simulink model "TST_CEngDsT_VD"  (R2016b)
settings: Solver=FixedStepDiscrete  StartTime=0.0  StopTime=simTime  FixedStep=sampleTime  RelTol=1e-3
values from neighbouring files (symbols this model uses):
  testCase = 1    [initTST_CEngDsT_VD_001.m]    (also in initTST_CEngDsT_VD_002.m = 2; initTST_CEngDsT_VD_003.m = 3; initTST_CEngDsT_VD_004.m = 4)
libraries: simulink x9, UnitTest_Lib x6
settings Model: Creator=dulinggang  LastModifiedBy=dulinggang
settings DebuggingCC: SignalRangeChecking=error

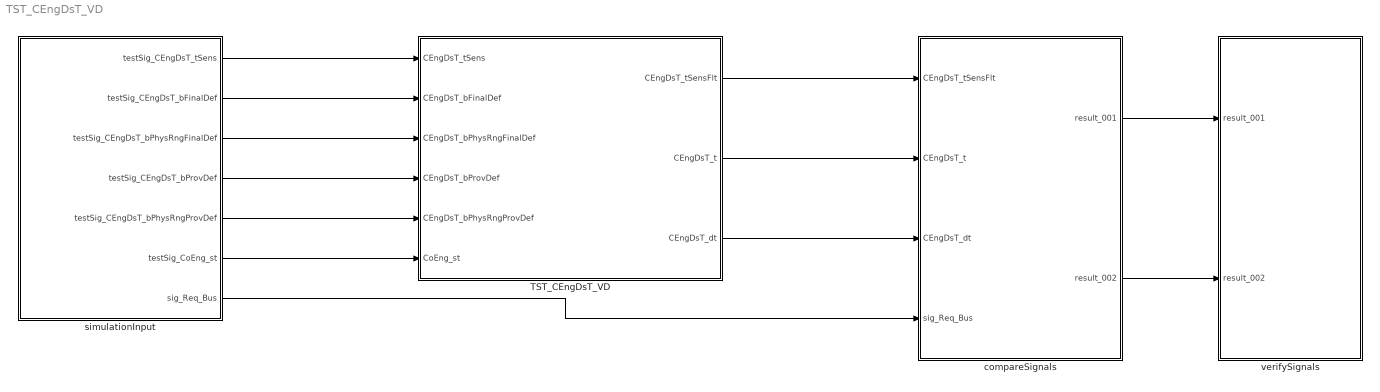
== system TST_CEngDsT_VD ==
  TST_CEngDsT_VD : Subsystem
  compareSignals : Subsystem
  simulationInput : Subsystem
  verifySignals : Subsystem
  wires:
  simulationInput/1(testSig_CEngDsT_tSens) -> TST_CEngDsT_VD/1(CEngDsT_tSens)
  simulationInput/2(testSig_CEngDsT_bFinalDef) -> TST_CEngDsT_VD/2(CEngDsT_bFinalDef)
  simulationInput/3(testSig_CEngDsT_bPhysRngFinalDef) -> TST_CEngDsT_VD/3(CEngDsT_bPhysRngFinalDef)
  simulationInput/4(testSig_CEngDsT_bProvDef) -> TST_CEngDsT_VD/4(CEngDsT_bProvDef)
  simulationInput/5(testSig_CEngDsT_bPhysRngProvDef) -> TST_CEngDsT_VD/5(CEngDsT_bPhysRngProvDef)
  simulationInput/6(testSig_CoEng_st) -> TST_CEngDsT_VD/6(CoEng_st)
  TST_CEngDsT_VD/1(CEngDsT_tSensFlt) -> compareSignals/1(CEngDsT_tSensFlt)
  TST_CEngDsT_VD/2(CEngDsT_t) -> compareSignals/2(CEngDsT_t)
  TST_CEngDsT_VD/3(CEngDsT_dt) -> compareSignals/3(CEngDsT_dt)
  simulationInput/7(sig_Req_Bus) -> compareSignals/4(sig_Req_Bus)
  compareSignals/1(result_001) -> verifySignals/1(result_001)
  compareSignals/2(result_002) -> verifySignals/2(result_002)

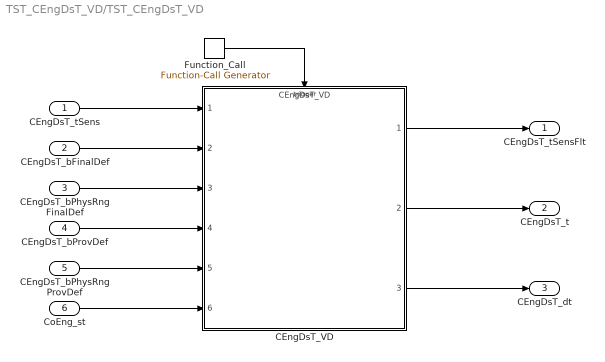
== system TST_CEngDsT_VD/TST_CEngDsT_VD ==
  CEngDsT_tSens : Inport
  CEngDsT_bFinalDef : Inport  Port=2
  CEngDsT_bPhysRngFinalDef : Inport  Port=3
  CEngDsT_bProvDef : Inport  Port=4
  CEngDsT_bPhysRngProvDef : Inport  Port=5
  CoEng_st : Inport  Port=6
  CEngDsT_VD : ModelReference  ModelNameDialog=CEngDsT_VD  SimulationMode=Normal  ModelReferenceVersion=1.125  TriggerPortName=function  TriggerPortTriggerType=function-call  TriggerPortStatesWhenEnabling=held
  Function_Call : simulink/Ports & Subsystems/Function-Call Generator  sample_time=sampleTime  numberOfIterations=1
  CEngDsT_tSensFlt : Outport
  CEngDsT_t : Outport  Port=2
  CEngDsT_dt : Outport  Port=3
  wires:
  Function_Call/1 -> CEngDsT_VD/Trigger
  CEngDsT_tSens/1 -> CEngDsT_VD/1
  CEngDsT_bFinalDef/1 -> CEngDsT_VD/2
  CEngDsT_bPhysRngFinalDef/1 -> CEngDsT_VD/3
  CEngDsT_bProvDef/1 -> CEngDsT_VD/4
  CEngDsT_bPhysRngProvDef/1 -> CEngDsT_VD/5
  CoEng_st/1 -> CEngDsT_VD/6
  CEngDsT_VD/1 -> CEngDsT_tSensFlt/1
  CEngDsT_VD/2 -> CEngDsT_t/1
  CEngDsT_VD/3 -> CEngDsT_dt/1

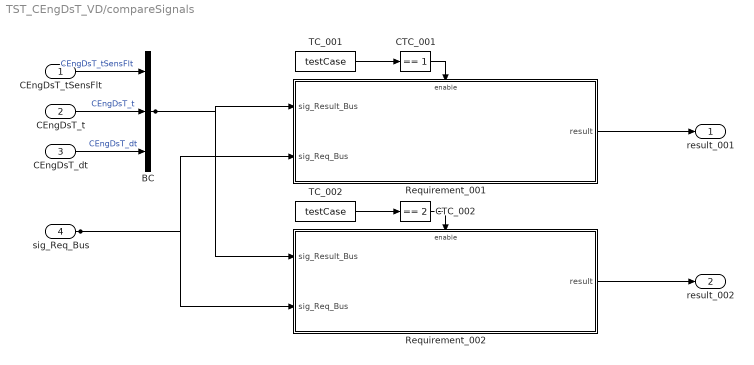
== system TST_CEngDsT_VD/compareSignals ==
  CEngDsT_tSensFlt : Inport
  CEngDsT_t : Inport  Port=2
  CEngDsT_dt : Inport  Port=3
  sig_Req_Bus : Inport  Port=4
  BC : BusCreator  Inputs=3
  CTC_001 : simulink/Logic and Bit Operations/Compare To Constant  relop===  const=1  OutDataTypeStr=boolean
  CTC_002 : simulink/Logic and Bit Operations/Compare To Constant  relop===  const=2  OutDataTypeStr=boolean
  Requirement_001 : Subsystem
  Requirement_002 : Subsystem
  TC_001 : Constant  Value=testCase
  TC_002 : Constant  Value=testCase
  result_001 : Outport
  result_002 : Outport  Port=2
  wires:
  CEngDsT_tSensFlt/1 -> BC/1  "CEngDsT_tSensFlt"
  CEngDsT_t/1 -> BC/2  "CEngDsT_t"
  CEngDsT_dt/1 -> BC/3  "CEngDsT_dt"
  TC_001/1 -> CTC_001/1
  CTC_001/1 -> Requirement_001/Enable
  sig_Req_Bus/1 -> Requirement_001/2(sig_Req_Bus), Requirement_002/2(sig_Req_Bus)
  BC/1 -> Requirement_001/1(sig_Result_Bus), Requirement_002/1(sig_Result_Bus)
  Requirement_001/1(result) -> result_001/1
  TC_002/1 -> CTC_002/1
  CTC_002/1 -> Requirement_002/Enable
  Requirement_002/1(result) -> result_002/1

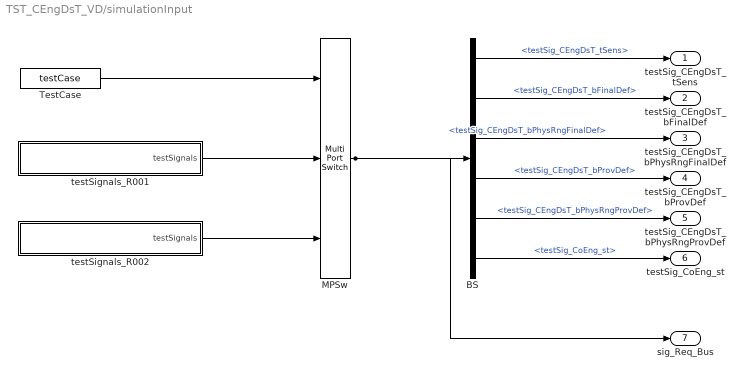
== system TST_CEngDsT_VD/simulationInput ==
  BS : BusSelector  OutputSignals=testSig_CEngDsT_tSens,testSig_CEngDsT_bFinalDef,testSig_CEngDsT_bPhysRngFinalDef,testSig_CEngDsT_bProvDef,testSig_CEngDsT_bPhysRngProvDef,testSig_CoEng_st
  MPSw : MultiPortSwitch  Inputs=2  SaturateOnIntegerOverflow=on  InputSameDT=on
  TestCase : Constant  Value=testCase
  testSignals_R001 : Subsystem
  testSignals_R002 : Subsystem
  testSig_CEngDsT_tSens : Outport
  testSig_CEngDsT_bFinalDef : Outport  Port=2
  testSig_CEngDsT_bPhysRngFinalDef : Outport  Port=3
  testSig_CEngDsT_bProvDef : Outport  Port=4
  testSig_CEngDsT_bPhysRngProvDef : Outport  Port=5
  testSig_CoEng_st : Outport  Port=6
  sig_Req_Bus : Outport  Port=7
  wires:
  BS/1 -> testSig_CEngDsT_tSens/1  "<testSig_CEngDsT_tSens>"
  BS/2 -> testSig_CEngDsT_bFinalDef/1  "<testSig_CEngDsT_bFinalDef>"
  BS/3 -> testSig_CEngDsT_bPhysRngFinalDef/1  "<testSig_CEngDsT_bPhysRngFinalDef>"
  BS/4 -> testSig_CEngDsT_bProvDef/1  "<testSig_CEngDsT_bProvDef>"
  BS/5 -> testSig_CEngDsT_bPhysRngProvDef/1  "<testSig_CEngDsT_bPhysRngProvDef>"
  BS/6 -> testSig_CoEng_st/1  "<testSig_CoEng_st>"
  MPSw/1 -> BS/1, sig_Req_Bus/1
  TestCase/1 -> MPSw/1
  testSignals_R001/1(testSignals) -> MPSw/2
  testSignals_R002/1(testSignals) -> MPSw/3

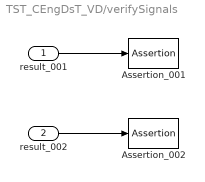
== system TST_CEngDsT_VD/verifySignals ==
  result_001 : Inport
  result_002 : Inport  Port=2
  Assertion_001 : Assertion  Enabled=off
  Assertion_002 : Assertion  Enabled=off
  wires:
  result_001/1 -> Assertion_001/1
  result_002/1 -> Assertion_002/1

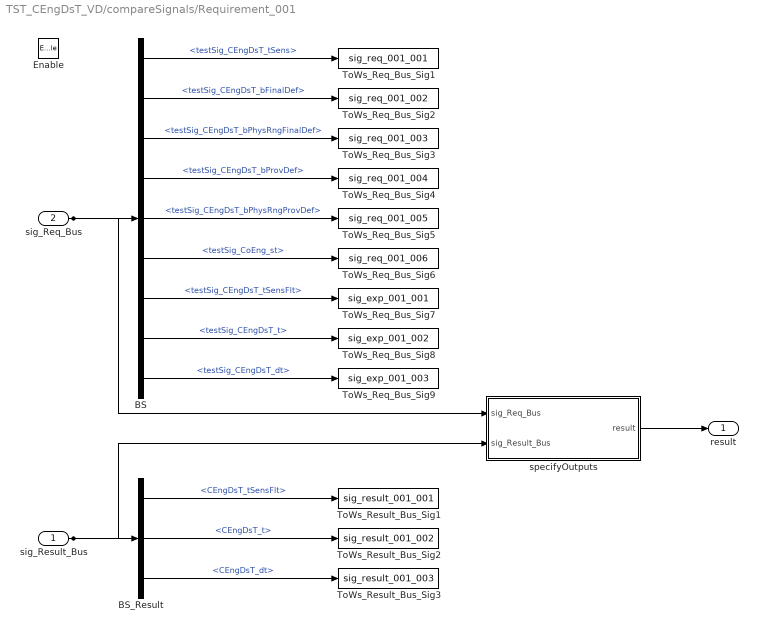
== system TST_CEngDsT_VD/compareSignals/Requirement_001 ==
  sig_Result_Bus : Inport
  sig_Req_Bus : Inport  Port=2
  Enable : EnablePort
  BS : BusSelector  OutputSignals=testSig_CEngDsT_tSens,testSig_CEngDsT_bFinalDef,testSig_CEngDsT_bPhysRngFinalDef,testSig_CEngDsT_bProvDef,testSig_CEngDsT_bPhysRngProvDef,testSig_CoEng_st,testSig_CEngDsT_tSensFlt,testSig_CEngDsT_t,testSig_CEngDsT_dt
  BS_Result : BusSelector  OutputSignals=CEngDsT_tSensFlt,CEngDsT_t,CEngDsT_dt
  ToWs_Req_Bus_Sig1 : ToWorkspace  VariableName=sig_req_001_001  SaveFormat=Structure With Time
  ToWs_Req_Bus_Sig2 : ToWorkspace  VariableName=sig_req_001_002  SaveFormat=Structure With Time
  ToWs_Req_Bus_Sig3 : ToWorkspace  VariableName=sig_req_001_003  SaveFormat=Structure With Time
  ToWs_Req_Bus_Sig4 : ToWorkspace  VariableName=sig_req_001_004  SaveFormat=Structure With Time
  ToWs_Req_Bus_Sig5 : ToWorkspace  VariableName=sig_req_001_005  SaveFormat=Structure With Time
  ToWs_Req_Bus_Sig6 : ToWorkspace  VariableName=sig_req_001_006  SaveFormat=Structure With Time
  ToWs_Req_Bus_Sig7 : ToWorkspace  VariableName=sig_exp_001_001  SaveFormat=Structure With Time
  ToWs_Req_Bus_Sig8 : ToWorkspace  VariableName=sig_exp_001_002  SaveFormat=Structure With Time
  ToWs_Req_Bus_Sig9 : ToWorkspace  VariableName=sig_exp_001_003  SaveFormat=Structure With Time
  ToWs_Result_Bus_Sig1 : ToWorkspace  VariableName=sig_result_001_001  SaveFormat=Structure With Time
  ToWs_Result_Bus_Sig2 : ToWorkspace  VariableName=sig_result_001_002  SaveFormat=Structure With Time
  ToWs_Result_Bus_Sig3 : ToWorkspace  VariableName=sig_result_001_003  SaveFormat=Structure With Time
  specifyOutputs : Subsystem
  result : Outport
  wires:
  sig_Req_Bus/1 -> BS/1, specifyOutputs/1(sig_Req_Bus)
  BS/1 -> ToWs_Req_Bus_Sig1/1  "<testSig_CEngDsT_tSens>"
  BS/2 -> ToWs_Req_Bus_Sig2/1  "<testSig_CEngDsT_bFinalDef>"
  BS/3 -> ToWs_Req_Bus_Sig3/1  "<testSig_CEngDsT_bPhysRngFinalDef>"
  BS/4 -> ToWs_Req_Bus_Sig4/1  "<testSig_CEngDsT_bProvDef>"
  BS/5 -> ToWs_Req_Bus_Sig5/1  "<testSig_CEngDsT_bPhysRngProvDef>"
  BS/6 -> ToWs_Req_Bus_Sig6/1  "<testSig_CoEng_st>"
  BS/7 -> ToWs_Req_Bus_Sig7/1  "<testSig_CEngDsT_tSensFlt>"
  BS/8 -> ToWs_Req_Bus_Sig8/1  "<testSig_CEngDsT_t>"
  BS/9 -> ToWs_Req_Bus_Sig9/1  "<testSig_CEngDsT_dt>"
  sig_Result_Bus/1 -> BS_Result/1, specifyOutputs/2(sig_Result_Bus)
  BS_Result/1 -> ToWs_Result_Bus_Sig1/1  "<CEngDsT_tSensFlt>"
  BS_Result/2 -> ToWs_Result_Bus_Sig2/1  "<CEngDsT_t>"
  BS_Result/3 -> ToWs_Result_Bus_Sig3/1  "<CEngDsT_dt>"
  specifyOutputs/1(result) -> result/1

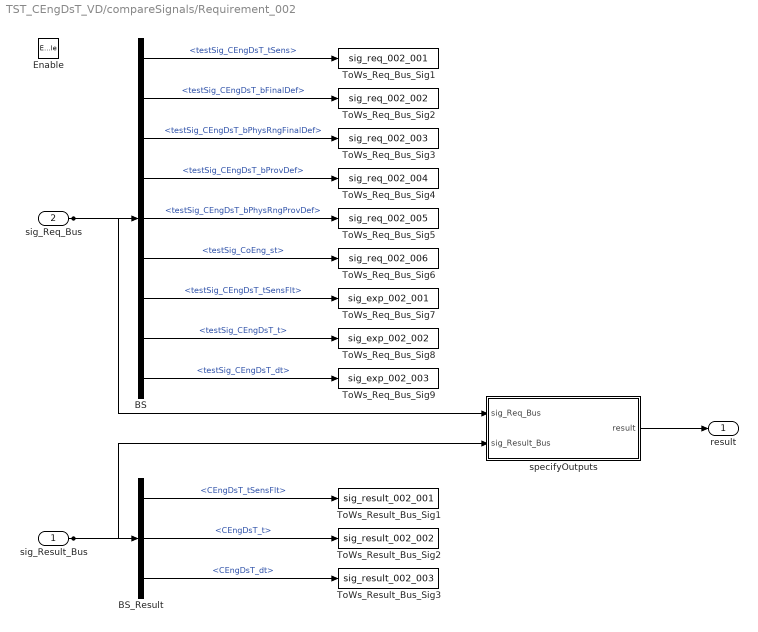
== system TST_CEngDsT_VD/compareSignals/Requirement_002 ==
  sig_Result_Bus : Inport
  sig_Req_Bus : Inport  Port=2
  Enable : EnablePort
  BS : BusSelector  OutputSignals=testSig_CEngDsT_tSens,testSig_CEngDsT_bFinalDef,testSig_CEngDsT_bPhysRngFinalDef,testSig_CEngDsT_bProvDef,testSig_CEngDsT_bPhysRngProvDef,testSig_CoEng_st,testSig_CEngDsT_tSensFlt,testSig_CEngDsT_t,testSig_CEngDsT_dt
  BS_Result : BusSelector  OutputSignals=CEngDsT_tSensFlt,CEngDsT_t,CEngDsT_dt
  ToWs_Req_Bus_Sig1 : ToWorkspace  VariableName=sig_req_002_001  SaveFormat=Structure With Time
  ToWs_Req_Bus_Sig2 : ToWorkspace  VariableName=sig_req_002_002  SaveFormat=Structure With Time
  ToWs_Req_Bus_Sig3 : ToWorkspace  VariableName=sig_req_002_003  SaveFormat=Structure With Time
  ToWs_Req_Bus_Sig4 : ToWorkspace  VariableName=sig_req_002_004  SaveFormat=Structure With Time
  ToWs_Req_Bus_Sig5 : ToWorkspace  VariableName=sig_req_002_005  SaveFormat=Structure With Time
  ToWs_Req_Bus_Sig6 : ToWorkspace  VariableName=sig_req_002_006  SaveFormat=Structure With Time
  ToWs_Req_Bus_Sig7 : ToWorkspace  VariableName=sig_exp_002_001  SaveFormat=Structure With Time
  ToWs_Req_Bus_Sig8 : ToWorkspace  VariableName=sig_exp_002_002  SaveFormat=Structure With Time
  ToWs_Req_Bus_Sig9 : ToWorkspace  VariableName=sig_exp_002_003  SaveFormat=Structure With Time
  ToWs_Result_Bus_Sig1 : ToWorkspace  VariableName=sig_result_002_001  SaveFormat=Structure With Time
  ToWs_Result_Bus_Sig2 : ToWorkspace  VariableName=sig_result_002_002  SaveFormat=Structure With Time
  ToWs_Result_Bus_Sig3 : ToWorkspace  VariableName=sig_result_002_003  SaveFormat=Structure With Time
  specifyOutputs : Subsystem
  result : Outport
  wires:
  sig_Req_Bus/1 -> BS/1, specifyOutputs/1(sig_Req_Bus)
  BS/1 -> ToWs_Req_Bus_Sig1/1  "<testSig_CEngDsT_tSens>"
  BS/2 -> ToWs_Req_Bus_Sig2/1  "<testSig_CEngDsT_bFinalDef>"
  BS/3 -> ToWs_Req_Bus_Sig3/1  "<testSig_CEngDsT_bPhysRngFinalDef>"
  BS/4 -> ToWs_Req_Bus_Sig4/1  "<testSig_CEngDsT_bProvDef>"
  BS/5 -> ToWs_Req_Bus_Sig5/1  "<testSig_CEngDsT_bPhysRngProvDef>"
  BS/6 -> ToWs_Req_Bus_Sig6/1  "<testSig_CoEng_st>"
  BS/7 -> ToWs_Req_Bus_Sig7/1  "<testSig_CEngDsT_tSensFlt>"
  BS/8 -> ToWs_Req_Bus_Sig8/1  "<testSig_CEngDsT_t>"
  BS/9 -> ToWs_Req_Bus_Sig9/1  "<testSig_CEngDsT_dt>"
  sig_Result_Bus/1 -> BS_Result/1, specifyOutputs/2(sig_Result_Bus)
  BS_Result/1 -> ToWs_Result_Bus_Sig1/1  "<CEngDsT_tSensFlt>"
  BS_Result/2 -> ToWs_Result_Bus_Sig2/1  "<CEngDsT_t>"
  BS_Result/3 -> ToWs_Result_Bus_Sig3/1  "<CEngDsT_dt>"
  specifyOutputs/1(result) -> result/1

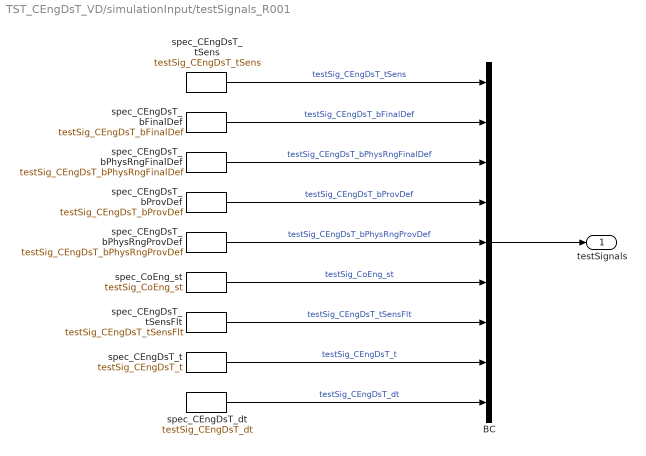
== system TST_CEngDsT_VD/simulationInput/testSignals_R001 ==
  BC : BusCreator  Inputs=9
  spec_CEngDsT_bFinalDef : FromWorkspace  VariableName=testSig_CEngDsT_bFinalDef  Interpolate=off  OutputAfterFinalValue=Holding final value
  spec_CEngDsT_bPhysRngFinalDef : FromWorkspace  VariableName=testSig_CEngDsT_bPhysRngFinalDef  Interpolate=off  OutputAfterFinalValue=Holding final value
  spec_CEngDsT_bPhysRngProvDef : FromWorkspace  VariableName=testSig_CEngDsT_bPhysRngProvDef  Interpolate=off  OutputAfterFinalValue=Holding final value
  spec_CEngDsT_bProvDef : FromWorkspace  VariableName=testSig_CEngDsT_bProvDef  Interpolate=off  OutputAfterFinalValue=Holding final value
  spec_CEngDsT_dt : FromWorkspace  VariableName=testSig_CEngDsT_dt  Interpolate=off  OutputAfterFinalValue=Holding final value
  spec_CEngDsT_t : FromWorkspace  VariableName=testSig_CEngDsT_t  Interpolate=off  OutputAfterFinalValue=Holding final value
  spec_CEngDsT_tSens : FromWorkspace  VariableName=testSig_CEngDsT_tSens  Interpolate=off  OutputAfterFinalValue=Holding final value
  spec_CEngDsT_tSensFlt : FromWorkspace  VariableName=testSig_CEngDsT_tSensFlt  Interpolate=off  OutputAfterFinalValue=Holding final value
  spec_CoEng_st : FromWorkspace  VariableName=testSig_CoEng_st  Interpolate=off  OutputAfterFinalValue=Holding final value
  testSignals : Outport
  wires:
  BC/1 -> testSignals/1
  spec_CEngDsT_tSens/1 -> BC/1  "testSig_CEngDsT_tSens"
  spec_CEngDsT_bFinalDef/1 -> BC/2  "testSig_CEngDsT_bFinalDef"
  spec_CEngDsT_bPhysRngFinalDef/1 -> BC/3  "testSig_CEngDsT_bPhysRngFinalDef"
  spec_CEngDsT_bProvDef/1 -> BC/4  "testSig_CEngDsT_bProvDef"
  spec_CEngDsT_bPhysRngProvDef/1 -> BC/5  "testSig_CEngDsT_bPhysRngProvDef"
  spec_CoEng_st/1 -> BC/6  "testSig_CoEng_st"
  spec_CEngDsT_tSensFlt/1 -> BC/7  "testSig_CEngDsT_tSensFlt"
  spec_CEngDsT_t/1 -> BC/8  "testSig_CEngDsT_t"
  spec_CEngDsT_dt/1 -> BC/9  "testSig_CEngDsT_dt"

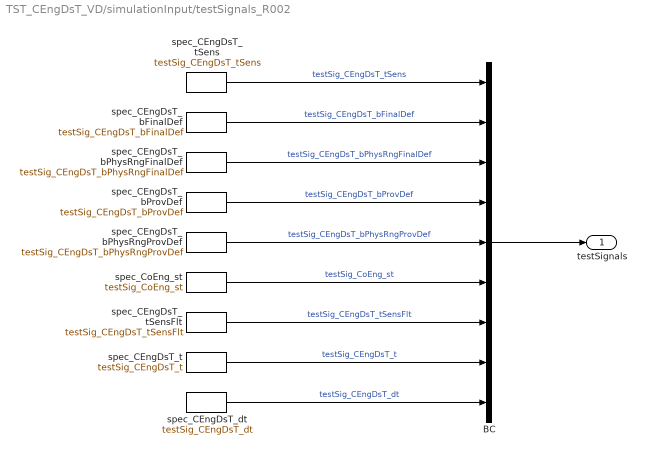
== system TST_CEngDsT_VD/simulationInput/testSignals_R002 ==
  BC : BusCreator  Inputs=9
  spec_CEngDsT_bFinalDef : FromWorkspace  VariableName=testSig_CEngDsT_bFinalDef  Interpolate=off  OutputAfterFinalValue=Holding final value
  spec_CEngDsT_bPhysRngFinalDef : FromWorkspace  VariableName=testSig_CEngDsT_bPhysRngFinalDef  Interpolate=off  OutputAfterFinalValue=Holding final value
  spec_CEngDsT_bPhysRngProvDef : FromWorkspace  VariableName=testSig_CEngDsT_bPhysRngProvDef  Interpolate=off  OutputAfterFinalValue=Holding final value
  spec_CEngDsT_bProvDef : FromWorkspace  VariableName=testSig_CEngDsT_bProvDef  Interpolate=off  OutputAfterFinalValue=Holding final value
  spec_CEngDsT_dt : FromWorkspace  VariableName=testSig_CEngDsT_dt  Interpolate=off  OutputAfterFinalValue=Holding final value
  spec_CEngDsT_t : FromWorkspace  VariableName=testSig_CEngDsT_t  Interpolate=off  OutputAfterFinalValue=Holding final value
  spec_CEngDsT_tSens : FromWorkspace  VariableName=testSig_CEngDsT_tSens  Interpolate=off  OutputAfterFinalValue=Holding final value
  spec_CEngDsT_tSensFlt : FromWorkspace  VariableName=testSig_CEngDsT_tSensFlt  Interpolate=off  OutputAfterFinalValue=Holding final value
  spec_CoEng_st : FromWorkspace  VariableName=testSig_CoEng_st  Interpolate=off  OutputAfterFinalValue=Holding final value
  testSignals : Outport
  wires:
  BC/1 -> testSignals/1
  spec_CEngDsT_tSens/1 -> BC/1  "testSig_CEngDsT_tSens"
  spec_CEngDsT_bFinalDef/1 -> BC/2  "testSig_CEngDsT_bFinalDef"
  spec_CEngDsT_bPhysRngFinalDef/1 -> BC/3  "testSig_CEngDsT_bPhysRngFinalDef"
  spec_CEngDsT_bProvDef/1 -> BC/4  "testSig_CEngDsT_bProvDef"
  spec_CEngDsT_bPhysRngProvDef/1 -> BC/5  "testSig_CEngDsT_bPhysRngProvDef"
  spec_CoEng_st/1 -> BC/6  "testSig_CoEng_st"
  spec_CEngDsT_tSensFlt/1 -> BC/7  "testSig_CEngDsT_tSensFlt"
  spec_CEngDsT_t/1 -> BC/8  "testSig_CEngDsT_t"
  spec_CEngDsT_dt/1 -> BC/9  "testSig_CEngDsT_dt"

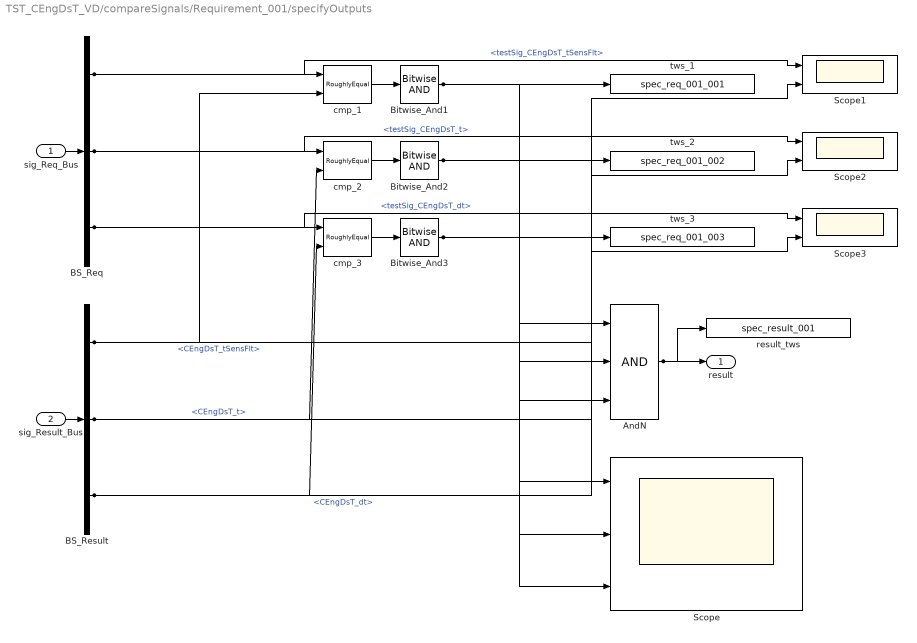
== system TST_CEngDsT_VD/compareSignals/Requirement_001/specifyOutputs ==
  sig_Req_Bus : Inport
  sig_Result_Bus : Inport  Port=2
  AndN : Logic  Inputs=3
  BS_Req : BusSelector  OutputSignals=testSig_CEngDsT_tSensFlt,testSig_CEngDsT_t,testSig_CEngDsT_dt
  BS_Result : BusSelector  OutputSignals=CEngDsT_tSensFlt,CEngDsT_t,CEngDsT_dt
  Bitwise_And1 : simulink/Logic and Bit Operations/Bitwise Operator  logicop=AND  UseBitMask=off  BitMask=bin2dec('11011001')  BitMaskRealWorld=Stored Integer
  Bitwise_And2 : simulink/Logic and Bit Operations/Bitwise Operator  logicop=AND  UseBitMask=off  BitMask=bin2dec('11011001')  BitMaskRealWorld=Stored Integer
  Bitwise_And3 : simulink/Logic and Bit Operations/Bitwise Operator  logicop=AND  UseBitMask=off  BitMask=bin2dec('11011001')  BitMaskRealWorld=Stored Integer
  Scope : Scope  NumInputPorts=3
  Scope1 : Scope  NumInputPorts=2
  Scope2 : Scope  NumInputPorts=2
  Scope3 : Scope  NumInputPorts=2
  cmp_1 : UnitTest_Lib/RoughlyEqual  slope=0.1
  cmp_2 : UnitTest_Lib/RoughlyEqual  slope=0.1
  cmp_3 : UnitTest_Lib/RoughlyEqual  slope=0.1
  result_tws : ToWorkspace  VariableName=spec_result_001
  tws_1 : ToWorkspace  VariableName=spec_req_001_001
  tws_2 : ToWorkspace  VariableName=spec_req_001_002
  tws_3 : ToWorkspace  VariableName=spec_req_001_003
  result : Outport
  wires:
  sig_Req_Bus/1 -> BS_Req/1
  sig_Result_Bus/1 -> BS_Result/1
  AndN/1 -> result/1, result_tws/1
  BS_Req/1 -> cmp_1/1, Scope1/1  "<testSig_CEngDsT_tSensFlt>"
  BS_Result/1 -> cmp_1/2, Scope1/2  "<CEngDsT_tSensFlt>"
  cmp_1/1 -> Bitwise_And1/1
  Bitwise_And1/1 -> tws_1/1, AndN/1, Scope/1
  BS_Req/2 -> cmp_2/1, Scope2/1  "<testSig_CEngDsT_t>"
  BS_Result/2 -> cmp_2/2, Scope2/2  "<CEngDsT_t>"
  cmp_2/1 -> Bitwise_And2/1
  Bitwise_And2/1 -> tws_2/1, AndN/2, Scope/2
  BS_Req/3 -> cmp_3/1, Scope3/1  "<testSig_CEngDsT_dt>"
  BS_Result/3 -> cmp_3/2, Scope3/2  "<CEngDsT_dt>"
  cmp_3/1 -> Bitwise_And3/1
  Bitwise_And3/1 -> tws_3/1, AndN/3, Scope/3

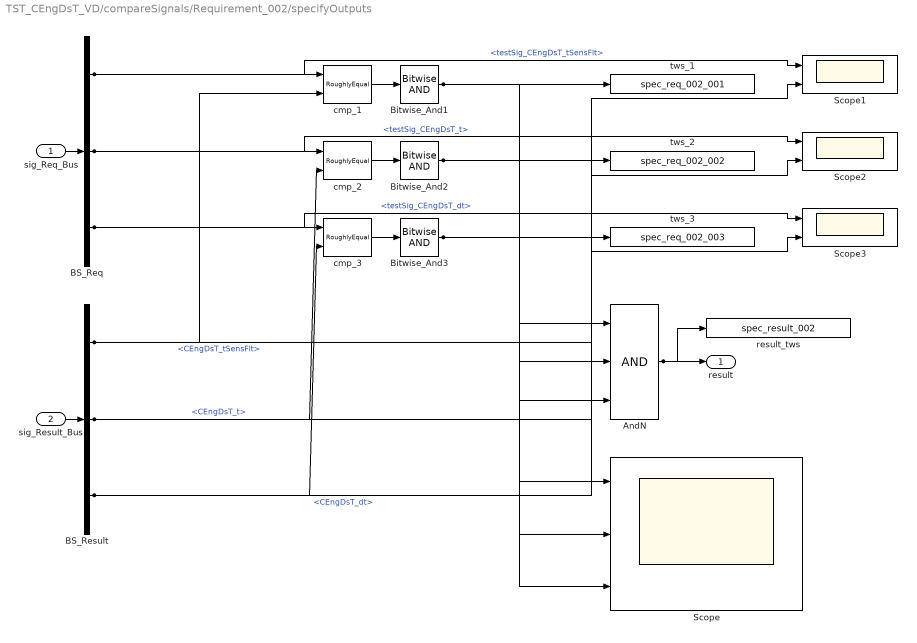
== system TST_CEngDsT_VD/compareSignals/Requirement_002/specifyOutputs ==
  sig_Req_Bus : Inport
  sig_Result_Bus : Inport  Port=2
  AndN : Logic  Inputs=3
  BS_Req : BusSelector  OutputSignals=testSig_CEngDsT_tSensFlt,testSig_CEngDsT_t,testSig_CEngDsT_dt
  BS_Result : BusSelector  OutputSignals=CEngDsT_tSensFlt,CEngDsT_t,CEngDsT_dt
  Bitwise_And1 : simulink/Logic and Bit Operations/Bitwise Operator  logicop=AND  UseBitMask=off  BitMask=bin2dec('11011001')  BitMaskRealWorld=Stored Integer
  Bitwise_And2 : simulink/Logic and Bit Operations/Bitwise Operator  logicop=AND  UseBitMask=off  BitMask=bin2dec('11011001')  BitMaskRealWorld=Stored Integer
  Bitwise_And3 : simulink/Logic and Bit Operations/Bitwise Operator  logicop=AND  UseBitMask=off  BitMask=bin2dec('11011001')  BitMaskRealWorld=Stored Integer
  Scope : Scope  NumInputPorts=3
  Scope1 : Scope  NumInputPorts=2
  Scope2 : Scope  NumInputPorts=2
  Scope3 : Scope  NumInputPorts=2
  cmp_1 : UnitTest_Lib/RoughlyEqual  slope=0.1
  cmp_2 : UnitTest_Lib/RoughlyEqual  slope=0.1
  cmp_3 : UnitTest_Lib/RoughlyEqual  slope=0.1
  result_tws : ToWorkspace  VariableName=spec_result_002
  tws_1 : ToWorkspace  VariableName=spec_req_002_001
  tws_2 : ToWorkspace  VariableName=spec_req_002_002
  tws_3 : ToWorkspace  VariableName=spec_req_002_003
  result : Outport
  wires:
  sig_Req_Bus/1 -> BS_Req/1
  sig_Result_Bus/1 -> BS_Result/1
  AndN/1 -> result/1, result_tws/1
  BS_Req/1 -> cmp_1/1, Scope1/1  "<testSig_CEngDsT_tSensFlt>"
  BS_Result/1 -> cmp_1/2, Scope1/2  "<CEngDsT_tSensFlt>"
  cmp_1/1 -> Bitwise_And1/1
  Bitwise_And1/1 -> tws_1/1, AndN/1, Scope/1
  BS_Req/2 -> cmp_2/1, Scope2/1  "<testSig_CEngDsT_t>"
  BS_Result/2 -> cmp_2/2, Scope2/2  "<CEngDsT_t>"
  cmp_2/1 -> Bitwise_And2/1
  Bitwise_And2/1 -> tws_2/1, AndN/2, Scope/2
  BS_Req/3 -> cmp_3/1, Scope3/1  "<testSig_CEngDsT_dt>"
  BS_Result/3 -> cmp_3/2, Scope3/2  "<CEngDsT_dt>"
  cmp_3/1 -> Bitwise_And3/1
  Bitwise_And3/1 -> tws_3/1, AndN/3, Scope/3
